simulink model "state_estimation_stress_test"  (R2016b)
settings: Solver=VariableStepAuto  StartTime=0.0  StopTime=200  RelTol=1e-3
values from neighbouring files (symbols this model uses):
  quat_cmd = quat_cmd/norm(quat_cmd)    [state_estimation_stress_test_init.m]    (also in state_estimation_test_init.m)
undefined symbols (not defined in the file or in its folder): fsw_params
libraries: dynamics_lib x2, pd_control_lib x1, sensors_lib x1, state_estimation x1, sensor_processing x1
settings Model: Creator=sexymathemagician  LastModifiedBy=sexymathemagician

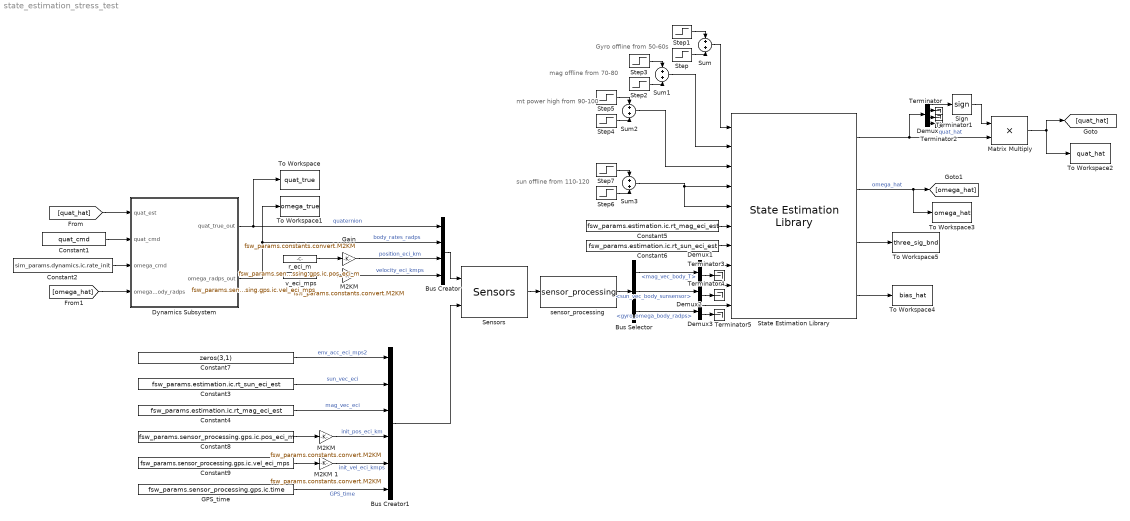
== system state_estimation_stress_test ==
  note: Gyro offline from 50-60s
  note: mag offline from 70-80
  note: mt power high from 90-100
  note: sun offline from 110-120
  Bus Creator : BusCreator  Inputs=4
  Bus Creator1 : BusCreator  Inputs=6
  Bus Selector : BusSelector  OutputSignals=mag_vec_body_T,sun_vec_body_sunsensor,gyro_omega_body_radps
  Constant1 : Constant  Value=quat_cmd
  Constant2 : Constant  Value=sim_params.dynamics.ic.rate_init
  Constant3 : Constant  Value=fsw_params.estimation.ic.rt_sun_eci_est
  Constant4 : Constant  Value=fsw_params.estimation.ic.rt_mag_eci_est
  Constant5 : Constant  Value=fsw_params.estimation.ic.rt_mag_eci_est
  Constant6 : Constant  Value=fsw_params.estimation.ic.rt_sun_eci_est
  Constant7 : Constant  Value=zeros(3,1)
  Constant8 : Constant  Value=fsw_params.sensor_processing.gps.ic.pos_eci_m
  Constant9 : Constant  Value=fsw_params.sensor_processing.gps.ic.vel_eci_mps
  Demux : Demux
  Demux1 : Demux  Outputs=[3 1]
  Demux2 : Demux  Outputs=[3 1]
  Demux3 : Demux  Outputs=[3 1]
  Dynamics Subsystem : Subsystem
  GPS_time : Constant  Value=fsw_params.sensor_processing.gps.ic.time
  Gain : Gain  Gain=fsw_params.constants.convert.M2KM
  M2KM : Gain  Gain=fsw_params.constants.convert.M2KM
  "M2KM " : Gain  Gain=fsw_params.constants.convert.M2KM
  M2KM 1 : Gain  Gain=fsw_params.constants.convert.M2KM
  Matrix Multiply : Product
  Sensors : sensors_lib/Sensors
      link override Bus Selector2: OutputSignals=sun_vec_eci,mag_vec_eci
  Sign : Signum
  State Estimation Library : state_estimation/State Estimation Library
  Step : Step  Time=50  Before=1  After=0  SampleTime=fsw_params.estimation.sample_time_s
  Step1 : Step  Time=60  SampleTime=fsw_params.estimation.sample_time_s
  Step2 : Step  Time=70  Before=1  After=0  SampleTime=fsw_params.estimation.sample_time_s
  Step3 : Step  Time=80  SampleTime=fsw_params.estimation.sample_time_s
  Step4 : Step  Time=90  Before=1  After=0  SampleTime=fsw_params.estimation.sample_time_s
  Step5 : Step  Time=100  SampleTime=fsw_params.estimation.sample_time_s
  Step6 : Step  Time=110  Before=1  After=0  SampleTime=fsw_params.estimation.sample_time_s
  Step7 : Step  Time=120  SampleTime=fsw_params.estimation.sample_time_s
  Sum{,1..3} (4 alike) : Sum
  Terminator{,1..5} (6 alike) : Terminator
  To Workspace : ToWorkspace  VariableName=quat_true  SaveFormat=Timeseries  SampleTime=-1
  To Workspace1 : ToWorkspace  VariableName=omega_true  SaveFormat=Timeseries  SampleTime=-1
  To Workspace2 : ToWorkspace  VariableName=quat_hat  SaveFormat=Timeseries  SampleTime=-1
  To Workspace3 : ToWorkspace  VariableName=omega_hat  SaveFormat=Timeseries  SampleTime=-1
  To Workspace4 : ToWorkspace  VariableName=bias_hat  SaveFormat=Timeseries  SampleTime=-1
  To Workspace5 : ToWorkspace  VariableName=three_sig_bnd  SaveFormat=Timeseries  SampleTime=-1
  r_eci_m : Constant  Value=fsw_params.sensor_processing.gps.ic.pos_eci_m
  sensor_processing : sensor_processing/sensor_processing
  v_eci_mps : Constant  Value=fsw_params.sensor_processing.gps.ic.vel_eci_mps
  wires:
  State Estimation Library/3 -> To Workspace5/1
  State Estimation Library/4 -> To Workspace4/1
  Dynamics Subsystem/1(quat_true_out) -> Bus Creator/1, To Workspace/1  "quaternion"
  Dynamics Subsystem/2(omega_radps_out) -> Bus Creator/2, To Workspace1/1  "body_rates_radps"
  [quat_hat] -> Dynamics Subsystem/1(quat_est)
  State Estimation Library/2 -> To Workspace3/1, [omega_hat]  "omega_hat"
  [omega_hat] -> Dynamics Subsystem/4(omega_body_radps)
  Constant1/1 -> Dynamics Subsystem/2(quat_cmd)
  Constant2/1 -> Dynamics Subsystem/3("omega_cmd ")
  State Estimation Library/1 -> Demux/1, Matrix Multiply/2  "quat_hat"
  Demux/2 -> Terminator/1
  Demux/3 -> Terminator1/1
  Demux/4 -> Terminator2/1
  Demux/1 -> Sign/1
  Sign/1 -> Matrix Multiply/1
  Sensors/1 -> sensor_processing/1
  sensor_processing/1 -> Bus Selector/1
  Bus Creator/1 -> Sensors/1
  Bus Selector/1 -> Demux1/1  "<mag_vec_body_T>"
  Bus Selector/2 -> Demux2/1  "<sun_vec_body_sunsensor>"
  Bus Selector/3 -> Demux3/1  "<gyro_omega_body_radps>"
  r_eci_m/1 -> Gain/1
  Constant4/1 -> Bus Creator1/3  "mag_vec_eci"
  Constant3/1 -> Bus Creator1/2  "sun_vec_eci"
  GPS_time/1 -> Bus Creator1/6  "GPS_time"
  Bus Creator1/1 -> Sensors/2
  Constant6/1 -> State Estimation Library/7
  Constant5/1 -> State Estimation Library/6
  Constant7/1 -> Bus Creator1/1  "env_acc_eci_mps2"
  Constant8/1 -> "M2KM "/1
  Constant9/1 -> M2KM 1/1
  Gain/1 -> Bus Creator/3  "position_eci_km"
  v_eci_mps/1 -> M2KM/1
  M2KM/1 -> Bus Creator/4  "velocity_eci_kmps"
  "M2KM "/1 -> Bus Creator1/4  "init_pos_eci_km"
  M2KM 1/1 -> Bus Creator1/5  "init_vel_eci_kmps"
  Demux1/1 -> State Estimation Library/8
  Demux2/1 -> State Estimation Library/9
  Demux3/1 -> State Estimation Library/10
  Demux1/2 -> Terminator3/1
  Demux2/2 -> Terminator4/1
  Demux3/2 -> Terminator5/1
  Matrix Multiply/1 -> To Workspace2/1, [quat_hat]
  Step1/1 -> Sum/1
  Step/1 -> Sum/2
  Sum/1 -> State Estimation Library/1
  Step3/1 -> Sum1/1
  Step2/1 -> Sum1/2
  Sum1/1 -> State Estimation Library/2
  Step5/1 -> Sum2/1
  Step4/1 -> Sum2/2
  Sum2/1 -> State Estimation Library/3
  Step7/1 -> Sum3/1
  Step6/1 -> Sum3/2
  Sum3/1 -> State Estimation Library/5, State Estimation Library/4

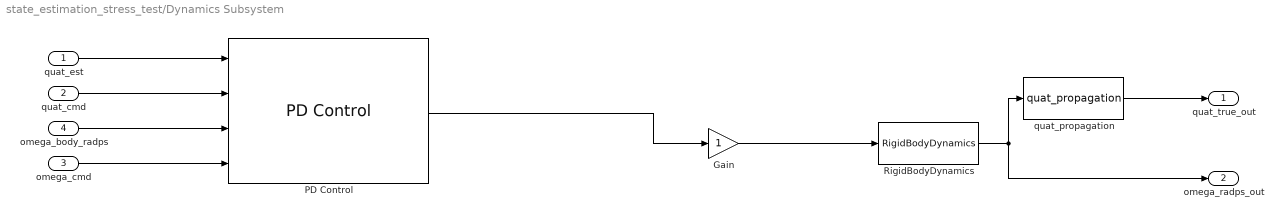
== system state_estimation_stress_test/Dynamics Subsystem ==
  quat_est : Inport
  quat_cmd : Inport  Port=2
  "omega_cmd " : Inport  Port=3
  omega_body_radps : Inport  Port=4
  Gain : Gain
  PD Control : pd_control_lib/PD Control
  RigidBodyDynamics : dynamics_lib/Dynamics/RigidBodyDynamics
  quat_propagation : dynamics_lib/Dynamics/quat_propagation
  quat_true_out : Outport
  omega_radps_out : Outport  Port=2
  wires:
  "omega_cmd "/1 -> PD Control/4
  quat_est/1 -> PD Control/1
  quat_cmd/1 -> PD Control/2
  omega_body_radps/1 -> PD Control/3
  RigidBodyDynamics/1 -> omega_radps_out/1, quat_propagation/1
  quat_propagation/1 -> quat_true_out/1
  PD Control/1 -> Gain/1
  Gain/1 -> RigidBodyDynamics/1
